simulink model "taylor_expansion_delayed_system"  (R2022a)
settings: Solver=ode4  StartTime=0.0  StopTime=200  FixedStep=1e-3  RelTol=1e-3
settings Model: Creator=manur  LastModifiedBy=manur

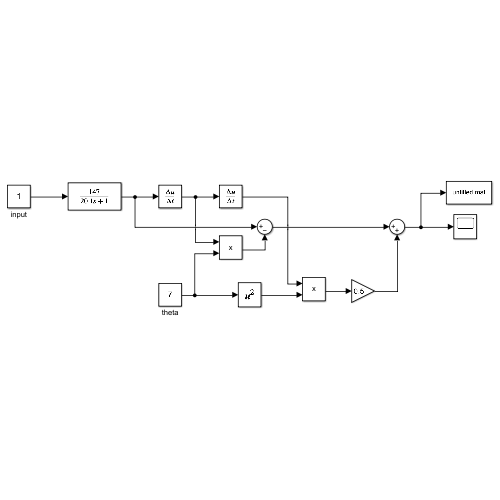
[thumbnail: Simulink's stored preview of the top-level diagram]
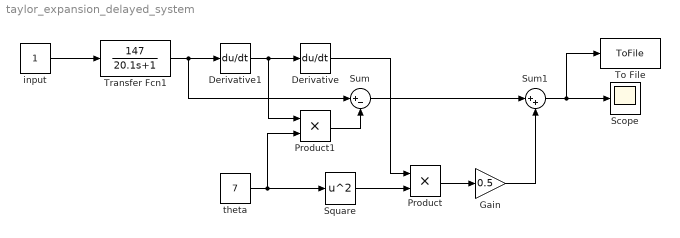
== system taylor_expansion_delayed_system ==
  Derivative : Derivative
  Derivative1 : Derivative
  Gain : Gain  Gain=0.5
  Product : Product
  Product1 : Product
  Scope : Scope
  Square : Math  Operator=square
  Sum : Sum  Inputs=|+-
  Sum1 : Sum  Inputs=|++
  To File : ToFile  SaveFormat=Timeseries
  Transfer Fcn1 : TransferFcn  Numerator=[147]  Denominator=[20.1 1]
  input : Constant
  theta : Constant  Value=7
  wires:
  Derivative1/1 -> Product1/1, Derivative/1
  Derivative/1 -> Product/1
  Square/1 -> Product/2
  theta/1 -> Square/1, Product1/2
  Product/1 -> Gain/1
  Product1/1 -> Sum/2
  Transfer Fcn1/1 -> Sum/1, Derivative1/1
  Gain/1 -> Sum1/2
  Sum/1 -> Sum1/1
  Sum1/1 -> Scope/1, To File/1
  input/1 -> Transfer Fcn1/1
